simulink model "Aircraft6dof_forTrimAndLin_ATT_wInputs"  (R2023b)
settings: Solver=ode4  StartTime=startTime  StopTime=stopTime  FixedStep=stepTime  RelTol=1e-3  EnableMultiTasking=on
values from neighbouring files (symbols this model uses):
  a0_s2 = 0    [SetupForTrimAndLin_Aircraft6dof.m]
  a0_s3 = 0    [SetupForTrimAndLin_Aircraft6dof.m]
  a0_s4 = 0.05    [SetupForTrimAndLin_Aircraft6dof.m]
  a0_s5 = 0.05    [SetupForTrimAndLin_Aircraft6dof.m]
  AR_s2 = b_s2 / c_s2    [SetupForTrimAndLin_Aircraft6dof.m]
  AR_s3 = b_s3 / c_s3    [SetupForTrimAndLin_Aircraft6dof.m]
  AR_s4 = (b_s4+b_s5) / c_s4    [SetupForTrimAndLin_Aircraft6dof.m]
  AR_s5 = (b_s4+b_s5) / c_s5    [SetupForTrimAndLin_Aircraft6dof.m]
  c_s2 = componentMassesAndGeom(3,2)    [SetupForTrimAndLin_Aircraft6dof.m]
  c_s3 = componentMassesAndGeom(4,2)    [SetupForTrimAndLin_Aircraft6dof.m]
  c_s4 = componentMassesAndGeom(1,2)    [SetupForTrimAndLin_Aircraft6dof.m]
  c_s5 = componentMassesAndGeom(2,2)    [SetupForTrimAndLin_Aircraft6dof.m]
  CD0_s2 = 0.01    [SetupForTrimAndLin_Aircraft6dof.m]
  CD0_s3 = 0.01    [SetupForTrimAndLin_Aircraft6dof.m]
  CD0_s4 = 0.01    [SetupForTrimAndLin_Aircraft6dof.m]
  CD0_s5 = 0.01    [SetupForTrimAndLin_Aircraft6dof.m]
  CDa_s2 = 1    [SetupForTrimAndLin_Aircraft6dof.m]
  CDa_s3 = 1    [SetupForTrimAndLin_Aircraft6dof.m]
  CDa_s4 = 1    [SetupForTrimAndLin_Aircraft6dof.m]
  CDa_s5 = 1    [SetupForTrimAndLin_Aircraft6dof.m]
  CL0_s2 = 0    [SetupForTrimAndLin_Aircraft6dof.m]
  CL0_s3 = 0    [SetupForTrimAndLin_Aircraft6dof.m]
  CL0_s4 = 0.05    [SetupForTrimAndLin_Aircraft6dof.m]
  CL0_s5 = 0.05    [SetupForTrimAndLin_Aircraft6dof.m]
  CM0_s2 = 0    [SetupForTrimAndLin_Aircraft6dof.m]
  CM0_s3 = 0    [SetupForTrimAndLin_Aircraft6dof.m]
  CM0_s4 = -0.05    [SetupForTrimAndLin_Aircraft6dof.m]
  CM0_s5 = -0.05    [SetupForTrimAndLin_Aircraft6dof.m]
  CMa_s2 = 0    [SetupForTrimAndLin_Aircraft6dof.m]
  CMa_s3 = 0    [SetupForTrimAndLin_Aircraft6dof.m]
  CMa_s4 = 0    [SetupForTrimAndLin_Aircraft6dof.m]
  CMa_s5 = 0    [SetupForTrimAndLin_Aircraft6dof.m]
  dCL_du = 3    [SetupForTrimAndLin_Aircraft6dof.m]
  dE_0 = 0    [SetupForTrimAndLin_Aircraft6dof.m]
  dEL_0 = 0    [SetupForTrimAndLin_Aircraft6dof.m]
  dER_0 = 0    [SetupForTrimAndLin_Aircraft6dof.m]
  dR_0 = 0    [SetupForTrimAndLin_Aircraft6dof.m]
  e_s2 = 0.8    [SetupForTrimAndLin_Aircraft6dof.m]
  e_s3 = 0.8    [SetupForTrimAndLin_Aircraft6dof.m]
  e_s4 = 0.9    [SetupForTrimAndLin_Aircraft6dof.m]
  e_s5 = 0.9    [SetupForTrimAndLin_Aircraft6dof.m]
  g_E_N = [0; 0; 9.81]*1    [SetupAndRun_Aircraft6dof.m]    (also in SetupForTrimAndLin_Aircraft6dof.m = [0; 0; 9.81])
  i_s2 = -0.1    [SetupForTrimAndLin_Aircraft6dof.m]
  i_s3 = 0    [SetupForTrimAndLin_Aircraft6dof.m]
  i_s4 = 0.0    (= 0)    [SetupForTrimAndLin_Aircraft6dof.m]
  i_s5 = 0.0    (= 0)    [SetupForTrimAndLin_Aircraft6dof.m]
  InitAtt = InitAtt_deg * deg2rad    [SetupAndRun_Aircraft6dof.m]    (also in SetupForTrimAndLin_Aircraft6dof.m)
  InitPos = InitPos_deg .* [deg2rad; deg2rad; 1]    [SetupAndRun_Aircraft6dof.m]    (also in SetupForTrimAndLin_Aircraft6dof.m)
  InitRates = Rates_Trim    [SetupAndRun_Aircraft6dof.m]    (also in SetupForTrimAndLin_Aircraft6dof.m = [0; 0; 0])
  InitVel = Vel_B_BA_Trim    [SetupAndRun_Aircraft6dof.m]    (also in SetupForTrimAndLin_Aircraft6dof.m = [15; 0; 0])
  J = zeros(3,3)    [DefineAircraftGeometry.m]    (also in InitializeModel.m = ASW.RotationalInertiaMatrix; SetupAndRun_Aircraft6dof.m = [0.049 0 -0.0004; 0 0.022 0; -0.0004 0 0.071]; SetupForTrimAndLin_Aircraft6dof.m)
  m = sum(obj.componentMassesAndGeom(:,1))    [DefineAircraftGeometry.m]    (also in SetupForTrimAndLin_Aircraft6dof.m = sum(componentMassesAndGeom(:,1)))
  MixMatrix = [-1 1 0 0 ... (first row only)    [SetupForTrimAndLin_Aircraft6dof.m]
  n_s2 = [0; 0; -1]    [SetupForTrimAndLin_Aircraft6dof.m]
  n_s3 = [0; 1; 0]    [SetupForTrimAndLin_Aircraft6dof.m]
  n_s4 = [0; sin(0*pi/180);  -cos(0*pi/180)]    [SetupForTrimAndLin_Aircraft6dof.m]
  n_s5 = [0; sin(0*pi/180);  -cos(0*pi/180)]    [SetupForTrimAndLin_Aircraft6dof.m]
  om_motor_init = 0    [SetupForTrimAndLin_Aircraft6dof.m]
  omDot_motor = 0    [SetupForTrimAndLin_Aircraft6dof.m]
  S_s2 = c_s2 * b_s2    [SetupForTrimAndLin_Aircraft6dof.m]
  S_s3 = c_s3 * b_s3    [SetupForTrimAndLin_Aircraft6dof.m]
  S_s4 = c_s4 * b_s4    [SetupForTrimAndLin_Aircraft6dof.m]
  S_s5 = c_s5 * b_s5    [SetupForTrimAndLin_Aircraft6dof.m]
  S_u_s2 = c_u_s2*b_s2    [SetupForTrimAndLin_Aircraft6dof.m]
  S_u_s3 = c_u_s3*b_s3    [SetupForTrimAndLin_Aircraft6dof.m]
  S_u_s4 = c_u_s4*b_s4    [SetupForTrimAndLin_Aircraft6dof.m]
  S_u_s5 = c_u_s5*b_s5    [SetupForTrimAndLin_Aircraft6dof.m]
  tauE = 0.1    [SetupForTrimAndLin_Aircraft6dof.m]
  tauEL = 0.1    [SetupForTrimAndLin_Aircraft6dof.m]
  tauER = 0.1    [SetupForTrimAndLin_Aircraft6dof.m]
  tauR = 0.1    [SetupForTrimAndLin_Aircraft6dof.m]
  v_N_AE = [0; 0; 0]    [SetupAndRun_Aircraft6dof.m]    (also in SetupForTrimAndLin_Aircraft6dof.m)
  x_cm = sum(obj.componentMassesAndGeom(:,1) .* obj.componentMassesAndGeom(:,5:7)) / m    [DefineAircraftGeometry.m]    (also in SetupForTrimAndLin_Aircraft6dof.m = x_cm')
  x_s2 = [componentMassesAndGeom(3,5) + (1/4)*componentMassesAndGeom(3,2); componentMassesAndGeom(3,6);componentMassesAndGeom(3,7)]    [SetupForTrimAndLin_Aircraft6dof.m]
  x_s3 = [componentMassesAndGeom(4,5) + (1/4)*componentMassesAndGeom(4,2); componentMassesAndGeom(4,6);componentMassesAndGeom(4,7)]    [SetupForTrimAndLin_Aircraft6dof.m]
  x_s4 = [componentMassesAndGeom(1,5) + (1/4)*componentMassesAndGeom(1,2); componentMassesAndGeom(1,6);componentMassesAndGeom(1,7)]    [SetupForTrimAndLin_Aircraft6dof.m]
  x_s5 = [componentMassesAndGeom(2,5) + (1/4)*componentMassesAndGeom(2,2); componentMassesAndGeom(2,6);componentMassesAndGeom(2,7)]    [SetupForTrimAndLin_Aircraft6dof.m]
undefined symbols (not defined in the file or in its folder): InitQuat, J_int, n_int
libraries: vrlib x7, simulink x3
(part 1 of 2)
settings Model: Creator=McArthur  LastModifiedBy=prafulsigdel
settings SolverCC: AlgebraicLoopSolver=TrustRegion
settings DataIOCC: InitialState=[]  LimitDataPoints=on  LoadInitialState=on  SaveFormat=StructureWithTime  ReturnWorkspaceOutputs=off
settings OptimizationCC: DefaultParameterBehavior=Inlined  BufferReuse=off  LifeSpan=inf
settings DebuggingCC: UnconnectedInputMsg=warning  UnconnectedOutputMsg=warning  UnconnectedLineMsg=warning  InitInArrayFormatMsg=none  SFUnexpectedBacktrackingDiag=warning  SFNoUnconditionalDefaultTransitionDiag=warning  SFExecutionAtInitializationDiag=none  ArithmeticOperatorsInVariantConditions=warning
settings HardwareCC: ProdBitPerSizeT=32  ProdBitPerPtrDiffT=32  ProdWordSize=32  ProdHWDeviceType=Specified
settings ModelReferenceCC: PropagateSignalLabelsOutOfModel=off
settings SFSimCC: SimUseLocalCustomCode=off  CustomCodeUndefinedFunction=UseInterfaceOnly
settings RTWCC: RTWUseLocalCustomCode=off
settings CodeAppCC: StateflowObjectComments=on
settings GRTTargetCC: TargetLangStandard=C89/C90 (ANSI)
settings ConfigComp: CovMetricSettings=dw  CovSaveCumulativeToWorkspaceVar=on  CovSaveSingleToWorkspaceVar=on  CovExternalEMLEnable=off

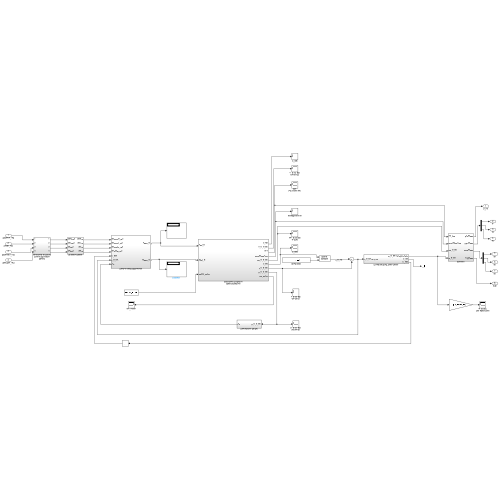
[thumbnail: Simulink's stored preview of the top-level diagram]
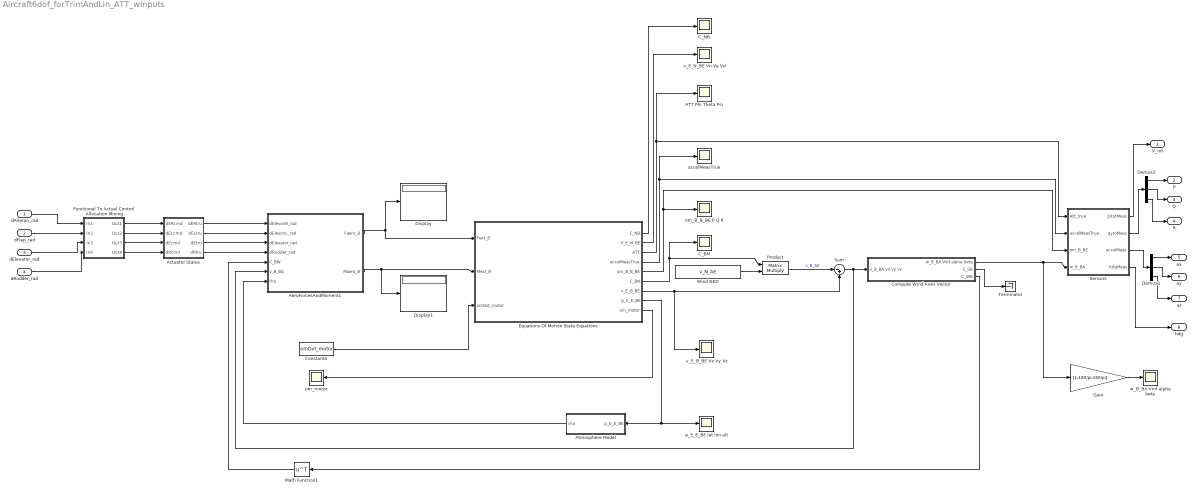
== system Aircraft6dof_forTrimAndLin_ATT_wInputs ==
  dAileron_rad : Inport
  dFlap_rad : Inport  Port=2
  dElevator_rad : Inport  Port=3
  dRudder_rad : Inport  Port=4
  ATT Phi Theta Psi : Scope
  Actuator States : Subsystem
  AeroForcesAndMoments : Subsystem
  Atmosphere Model : Subsystem
  C_BN : Scope
  C_NB : Scope
  Compute Wind Axes Vector : Subsystem
  Constant4 : Constant  Value=omDot_motor
  Demux1 : Demux  Outputs=3
  Demux2 : Demux  Outputs=3
  Display : Display
  Display1 : Display
  Equations Of Motion State Equations : Subsystem
  Functional To Actual Control Allocation Mixing : Subsystem
  Gain : Gain  Gain=[1;180/pi;180/pi]
  Math Function1 : Math  Operator=transpose  SignedPower=on
  Product : Product  Multiplication=Matrix(*)
  Sensors : Subsystem
  Sum : Sum  Inputs=|-+
  Terminator : Terminator
  Wind NED : Constant  Value=v_N_AE
  accelMeasTrue : Scope
  om_B_B_BE P Q R : Scope
  om_motor : Scope
  p_E_E_BE lat lon alt : Scope
  v_E_B_BE Vx Vy Vz : Scope
  v_E_N_BE Vn Ve Vd : Scope
  w_B_BA Vinf alpha beta : Scope
  V_inf : Outport
  P : Outport  Port=2
  Q : Outport  Port=3
  R : Outport  Port=4
  ax : Outport  Port=5
  ay : Outport  Port=6
  az : Outport  Port=7
  hdg : Outport  Port=8
  wires:
  Equations Of Motion State Equations/8(p_E_E_BE) -> Atmosphere Model/1(p_E_E_BE), p_E_E_BE lat lon alt/1
  Equations Of Motion State Equations/3(ATT) -> ATT Phi Theta Psi/1, Sensors/1(Att_true)
  AeroForcesAndMoments/2(Maero_B) -> Display1/1, Equations Of Motion State Equations/2(Mext_B)
  Constant4/1 -> Equations Of Motion State Equations/3(omDot_motor)
  AeroForcesAndMoments/1(Faero_B) -> Display/1, Equations Of Motion State Equations/1(Fext_B)
  Equations Of Motion State Equations/5(om_B_B_BE) -> Sensors/3(om_B_BE), om_B_B_BE P Q R/1
  Equations Of Motion State Equations/1(C_NB) -> C_NB/1
  Equations Of Motion State Equations/6(C_BN) -> C_BN/1, Product/1
  Equations Of Motion State Equations/7(v_E_B_BE) -> Sum/2, v_E_B_BE Vx Vy Vz/1
  Equations Of Motion State Equations/2(V_E_N_BE) -> v_E_N_BE Vn Ve Vd/1
  Compute Wind Axes Vector/1(w_B_BA Vinf alpha beta) -> Gain/1, Sensors/4(w_B_BA)
  Sum/1 -> AeroForcesAndMoments/6(v_B_BA), Compute Wind Axes Vector/1(v_B_BA vx vy vz)
  Product/1 -> Sum/1  "v_B_AE"
  Gain/1 -> w_B_BA Vinf alpha beta/1
  Equations Of Motion State Equations/9(om_motor) -> om_motor/1
  Atmosphere Model/1(rho) -> AeroForcesAndMoments/7(rho)
  Math Function1/1 -> AeroForcesAndMoments/5(C_BW)
  Compute Wind Axes Vector/3(C_WB) -> Math Function1/1
  Compute Wind Axes Vector/2(C_SB) -> Terminator/1
  Demux2/1 -> P/1
  Demux2/2 -> Q/1
  Demux2/3 -> R/1
  Sensors/1(pitotMeas) -> V_inf/1
  Sensors/2(gyroMeas) -> Demux2/1
  Equations Of Motion State Equations/4(accelMeasTrue) -> Sensors/2(accelMeasTrue), accelMeasTrue/1
  Wind NED/1 -> Product/2
  Demux1/1 -> ax/1
  Demux1/2 -> ay/1
  Demux1/3 -> az/1
  Sensors/3(accelMeas) -> Demux1/1
  Sensors/4(hdgMeas) -> hdg/1
  dAileron_rad/1 -> Functional To Actual Control Allocation Mixing/1(In1)
  dFlap_rad/1 -> Functional To Actual Control Allocation Mixing/2(In2)
  dElevator_rad/1 -> Functional To Actual Control Allocation Mixing/3(In3)
  dRudder_rad/1 -> Functional To Actual Control Allocation Mixing/4(In4)
  Functional To Actual Control Allocation Mixing/1(Out1) -> Actuator States/1(dERcmd)
  Functional To Actual Control Allocation Mixing/2(Out2) -> Actuator States/2(dELcmd)
  Functional To Actual Control Allocation Mixing/3(Out3) -> Actuator States/3(dEcmd)
  Functional To Actual Control Allocation Mixing/4(Out4) -> Actuator States/4(dRcmd)
  Actuator States/1(dERtru) -> AeroForcesAndMoments/1(dElevonR_rad)
  Actuator States/2(dELtru) -> AeroForcesAndMoments/2(dElevonL_rad)
  Actuator States/3(dEtru) -> AeroForcesAndMoments/3(dElevator_rad)
  Actuator States/4(dRtru) -> AeroForcesAndMoments/4(dRudder_rad)

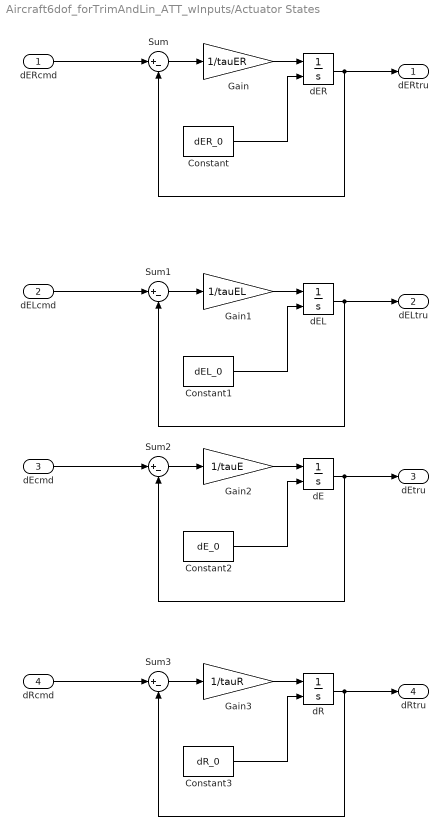
== system Aircraft6dof_forTrimAndLin_ATT_wInputs/Actuator States ==
  dERcmd : Inport
  dELcmd : Inport  Port=2
  dEcmd : Inport  Port=3
  dRcmd : Inport  Port=4
  Constant : Constant  Value=dER_0
  Constant1 : Constant  Value=dEL_0
  Constant2 : Constant  Value=dE_0
  Constant3 : Constant  Value=dR_0
  Gain : Gain  Gain=1/tauER
  Gain1 : Gain  Gain=1/tauEL
  Gain2 : Gain  Gain=1/tauE
  Gain3 : Gain  Gain=1/tauR
  Sum{,1..3} (4 alike) : Sum  Inputs=|+-
  dE : Integrator  InitialConditionSource=external
  dEL : Integrator  InitialConditionSource=external
  dER : Integrator  InitialConditionSource=external
  dR : Integrator  InitialConditionSource=external
  dERtru : Outport
  dELtru : Outport  Port=2
  dEtru : Outport  Port=3
  dRtru : Outport  Port=4
  wires:
  dER/1 -> Sum/2, dERtru/1
  dERcmd/1 -> Sum/1
  Gain/1 -> dER/1
  Sum/1 -> Gain/1
  Constant/1 -> dER/2
  dEL/1 -> Sum1/2, dELtru/1
  dELcmd/1 -> Sum1/1
  Gain1/1 -> dEL/1
  Sum1/1 -> Gain1/1
  Constant1/1 -> dEL/2
  dE/1 -> Sum2/2, dEtru/1
  dEcmd/1 -> Sum2/1
  Gain2/1 -> dE/1
  Sum2/1 -> Gain2/1
  Constant2/1 -> dE/2
  dR/1 -> Sum3/2, dRtru/1
  dRcmd/1 -> Sum3/1
  Gain3/1 -> dR/1
  Sum3/1 -> Gain3/1
  Constant3/1 -> dR/2

== system Aircraft6dof_forTrimAndLin_ATT_wInputs/AeroForcesAndMoments ==
  dElevonR_rad : Inport
  dElevonL_rad : Inport  Port=2
  dElevator_rad : Inport  Port=3
  dRudder_rad : Inport  Port=4
  C_BW : Inport  Port=5
  v_B_BA : Inport  Port=6
  rho : Inport  Port=7
  Add : Sum  Inputs=++++
  Add1 : Sum  Inputs=++++
  Display1 : Display
  Display3 : Display
  Surface2 : Subsystem
  Surface3 : Subsystem
  Surface4 : Subsystem
  Surface5 : Subsystem
  Faero_B : Outport
  Maero_B : Outport  Port=2
  wires:
  C_BW/1 -> Surface2/1(C_BW), Surface3/1(C_BW), Surface5/1(C_BW), Surface4/1(C_BW)
  v_B_BA/1 -> Surface3/2(v_B_BA), Surface2/2(v_B_BA), Surface5/2(v_B_BA), Surface4/2(v_B_BA)
  rho/1 -> Surface3/3(rho), Surface2/3(rho), Surface5/3(rho), Surface4/3(rho)
  Surface4/1(Fs4_B) -> Add/1
  Surface5/1(Fs5_B) -> Add/2
  Surface4/2(Ms4_B) -> Add1/1
  Surface5/2(Ms5_B) -> Add1/2
  Surface2/1(Fs2_B) -> Add/3
  Surface2/2(Ms2_B) -> Add1/3
  Add1/1 -> Display1/1, Maero_B/1
  Add/1 -> Display3/1, Faero_B/1
  Surface3/1(Fs2_B) -> Add/4
  Surface3/2(Ms2_B) -> Add1/4
  dElevonR_rad/1 -> Surface4/4(u_s#_rad)
  dElevonL_rad/1 -> Surface5/4(u_s#_rad)
  dElevator_rad/1 -> Surface2/4(u_s#_rad)
  dRudder_rad/1 -> Surface3/4(u_s#_rad)

== system Aircraft6dof_forTrimAndLin_ATT_wInputs/Atmosphere Model ==
  p_E_E_BE : Inport
  Compare To Constant : simulink/Logic and Bit Operations/Compare To Constant  relop=<=  const=11000  OutDataTypeStr=boolean
  Demux : Demux  Outputs=3
  Enhance Me Please! : Constant  Value=0
  Standard Atmosphere - Troposphere : MATLAB Function  TreatAsAtomicUnit=on
  Switch : Switch  Criteria=u2 ~= 0  Threshold=11000  SaturateOnIntegerOverflow=off  InputSameDT=off
  Terminator : Terminator
  Terminator1 : Terminator
  rho : Outport
  wires:
  p_E_E_BE/1 -> Demux/1
  Demux/1 -> Terminator/1
  Demux/2 -> Terminator1/1
  Demux/3 -> Standard Atmosphere - Troposphere/1(h), Compare To Constant/1
  Compare To Constant/1 -> Switch/2
  Standard Atmosphere - Troposphere/1(rho) -> Switch/1
  Switch/1 -> rho/1
  Enhance Me Please!/1 -> Switch/3

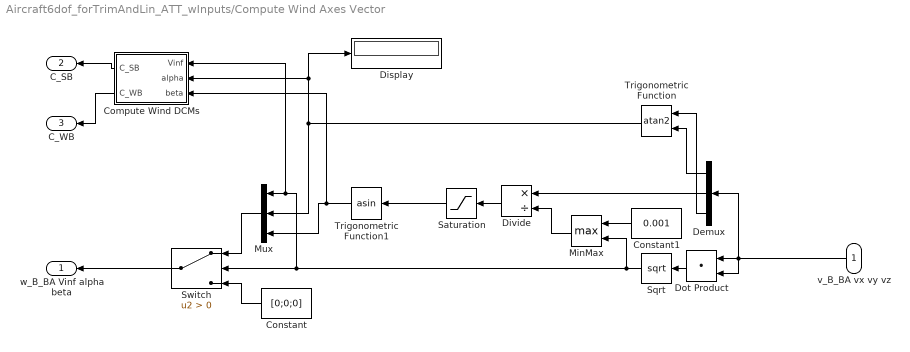
== system Aircraft6dof_forTrimAndLin_ATT_wInputs/Compute Wind Axes Vector ==
  v_B_BA vx vy vz : Inport
  Compute Wind DCMs : MATLAB Function  TreatAsAtomicUnit=on
  Constant : Constant  Value=[0;0;0]
  Constant1 : Constant  Value=0.001
  Demux : Demux  Outputs=3
  Display : Display
  Divide : Product  Inputs=*/
  Dot Product : DotProduct  OutDataTypeStr=Inherit: Inherit via internal rule
  MinMax : MinMax  Function=max  Inputs=2
  Mux : Mux  Inputs=3
  Saturation : Saturate  UpperLimit=1  LowerLimit=-1
  Sqrt : Sqrt
  Switch : Switch  Criteria=u2 > Threshold  SaturateOnIntegerOverflow=off  InputSameDT=off
  Trigonometric Function : Trigonometry  Operator=atan2
  Trigonometric Function1 : Trigonometry  Operator=asin
  w_B_BA Vinf alpha beta : Outport
  C_SB : Outport  Port=2
  C_WB : Outport  Port=3
  wires:
  Dot Product/1 -> Sqrt/1
  Mux/1 -> Switch/1
  Constant/1 -> Switch/3
  Trigonometric Function/1 -> Display/1, Compute Wind DCMs/2(alpha), Mux/2
  Switch/1 -> w_B_BA Vinf alpha beta/1
  Demux/3 -> Trigonometric Function/1
  v_B_BA vx vy vz/1 -> Demux/1, Dot Product/2, Dot Product/1
  Demux/1 -> Trigonometric Function/2
  Constant1/1 -> MinMax/1
  MinMax/1 -> Divide/2
  Demux/2 -> Divide/1
  Divide/1 -> Saturation/1
  Saturation/1 -> Trigonometric Function1/1
  Trigonometric Function1/1 -> Compute Wind DCMs/3(beta), Mux/3
  Sqrt/1 -> Compute Wind DCMs/1(Vinf), Mux/1, Switch/2, MinMax/2
  Compute Wind DCMs/2(C_WB) -> C_WB/1
  Compute Wind DCMs/1(C_SB) -> C_SB/1

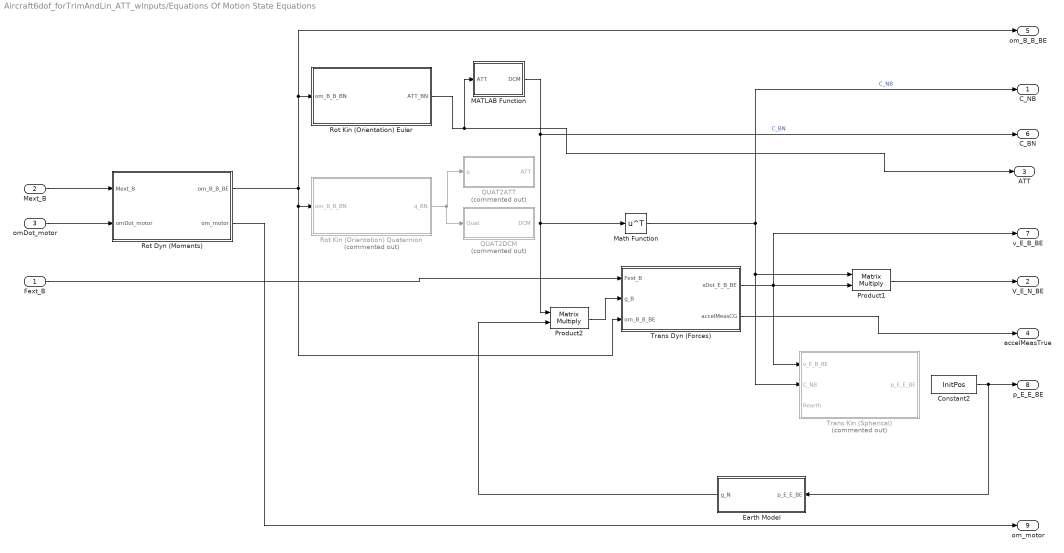
== system Aircraft6dof_forTrimAndLin_ATT_wInputs/Equations Of Motion State Equations ==
  Fext_B : Inport
  Mext_B : Inport  Port=2
  omDot_motor : Inport  Port=3
  Constant2 : Constant  Value=InitPos
  Earth Model : Subsystem
  MATLAB Function : MATLAB Function  TreatAsAtomicUnit=on
  Math Function : Math  Operator=transpose  SignedPower=on
  Product1 : Product  Multiplication=Matrix(*)
  Product2 : Product  Multiplication=Matrix(*)
  QUAT2ATT : Subsystem  Commented=on
  QUAT2DCM : Subsystem  Commented=on
  Rot Dyn (Moments) : Subsystem
  Rot Kin (Orientation) Euler : Subsystem
  Rot Kin (Orientation) Quaternion : Subsystem  Commented=on
  Trans Dyn (Forces) : Subsystem
  Trans Kin (Spherical) : Subsystem  Commented=on
  C_NB : Outport
  V_E_N_BE : Outport  Port=2
  ATT : Outport  Port=3
  accelMeasTrue : Outport  Port=4
  om_B_B_BE : Outport  Port=5
  C_BN : Outport  Port=6
  v_E_B_BE : Outport  Port=7
  p_E_E_BE : Outport  Port=8
  om_motor : Outport  Port=9
  wires:
  omDot_motor/1 -> Rot Dyn (Moments)/2(omDot_motor)
  Rot Dyn (Moments)/1(om_B_B_BE) -> Trans Dyn (Forces)/3(om_B_B_BE), Rot Kin (Orientation) Quaternion/1(om_B_B_BN), Rot Kin (Orientation) Euler/1(om_B_B_BN), om_B_B_BE/1
  Trans Dyn (Forces)/1(xDot_E_B_BE) -> Trans Kin (Spherical)/1(v_E_B_BE), v_E_B_BE/1, Product1/2
  Rot Kin (Orientation) Quaternion/1(q_BN) -> QUAT2DCM/1(Quat), QUAT2ATT/1(q)
  MATLAB Function/1(DCM) -> Math Function/1, Product2/1, C_BN/1  "C_BN"
  Mext_B/1 -> Rot Dyn (Moments)/1(Mext_B)
  Fext_B/1 -> Trans Dyn (Forces)/1(Fext_B)
  Rot Kin (Orientation) Euler/1(ATT_BN) -> ATT/1, MATLAB Function/1(ATT)
  Constant2/1 -> Earth Model/1(p_E_E_BE), p_E_E_BE/1
  Math Function/1 -> C_NB/1, Trans Kin (Spherical)/2(C_NB), Product1/1  "C_NB"
  Product1/1 -> V_E_N_BE/1
  Earth Model/1(g_N) -> Product2/2
  Product2/1 -> Trans Dyn (Forces)/2(g_B)
  Rot Dyn (Moments)/2(om_motor) -> om_motor/1
  Trans Dyn (Forces)/2(accelMeasCG) -> accelMeasTrue/1

== system Aircraft6dof_forTrimAndLin_ATT_wInputs/Functional To Actual Control Allocation Mixing ==
  In1 : Inport
  In2 : Inport  Port=2
  In3 : Inport  Port=3
  In4 : Inport  Port=4
  Constant1 : Constant  Value=MixMatrix
  Demux : Demux
  Mux : Mux
  Product1 : Product  Multiplication=Matrix(*)
  Out1 : Outport
  Out2 : Outport  Port=2
  Out3 : Outport  Port=3
  Out4 : Outport  Port=4
  wires:
  In1/1 -> Mux/1
  In2/1 -> Mux/2
  In3/1 -> Mux/3
  In4/1 -> Mux/4
  Demux/2 -> Out2/1
  Constant1/1 -> Product1/1
  Mux/1 -> Product1/2
  Demux/1 -> Out1/1
  Demux/4 -> Out4/1
  Demux/3 -> Out3/1
  Product1/1 -> Demux/1

== system Aircraft6dof_forTrimAndLin_ATT_wInputs/Sensors ==
  Att_true : Inport
  accelMeasTrue : Inport  Port=2
  om_B_BE : Inport  Port=3
  w_B_BA : Inport  Port=4
  Demux : Demux  Outputs=3
  Demux1 : Demux  Outputs=3
  Terminator{1..4} (4 alike) : Terminator
  pitotMeas : Outport
  gyroMeas : Outport  Port=2
  accelMeas : Outport  Port=3
  hdgMeas : Outport  Port=4
  wires:
  om_B_BE/1 -> gyroMeas/1
  w_B_BA/1 -> Demux/1
  Demux/3 -> Terminator1/1
  Demux/2 -> Terminator2/1
  Demux/1 -> pitotMeas/1
  accelMeasTrue/1 -> accelMeas/1
  Att_true/1 -> Demux1/1
  Demux1/1 -> Terminator3/1
  Demux1/2 -> Terminator4/1
  Demux1/3 -> hdgMeas/1

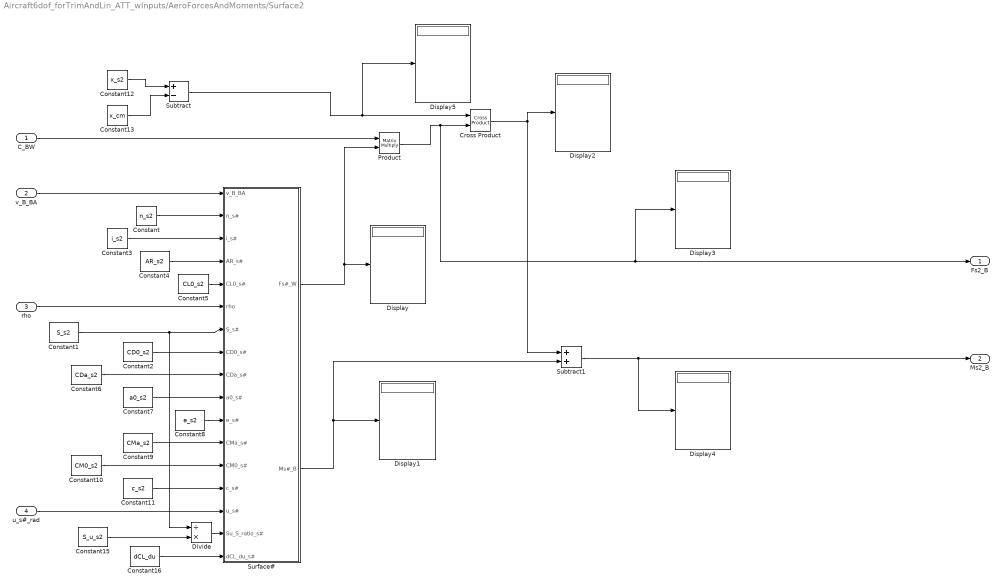
== system Aircraft6dof_forTrimAndLin_ATT_wInputs/AeroForcesAndMoments/Surface2 ==
  C_BW : Inport
  v_B_BA : Inport  Port=2
  rho : Inport  Port=3
  u_s#_rad : Inport  Port=4
  Constant : Constant  Value=n_s2
  Constant1 : Constant  Value=S_s2
  Constant10 : Constant  Value=CM0_s2
  Constant11 : Constant  Value=c_s2
  Constant12 : Constant  Value=x_s2
  Constant13 : Constant  Value=x_cm
  Constant15 : Constant  Value=S_u_s2
  Constant16 : Constant  Value=dCL_du
  Constant2 : Constant  Value=CD0_s2
  Constant3 : Constant  Value=i_s2
  Constant4 : Constant  Value=AR_s2
  Constant5 : Constant  Value=CL0_s2
  Constant6 : Constant  Value=CDa_s2
  Constant7 : Constant  Value=a0_s2
  Constant8 : Constant  Value=e_s2
  Constant9 : Constant  Value=CMa_s2
  Cross Product : vrlib/Utilities/Cross Product
  Display{,1..5} (6 alike) : Display
  Divide : Product  Inputs=/*
  Product : Product  Multiplication=Matrix(*)
  Subtract : Sum  Inputs=+-
  Subtract1 : Sum
  Surface# : Subsystem
  Fs2_B : Outport
  Ms2_B : Outport  Port=2
  wires:
  Subtract/1 -> Display5/1, Cross Product/1
  C_BW/1 -> Product/1
  Constant12/1 -> Subtract/1
  Constant13/1 -> Subtract/2
  Cross Product/1 -> Subtract1/1, Display2/1
  Product/1 -> Fs2_B/1, Display3/1, Cross Product/2
  Subtract1/1 -> Ms2_B/1, Display4/1
  Surface#/2(Ms#_B) -> Subtract1/2, Display1/1
  Constant10/1 -> Surface#/13(CM0_s#)
  Surface#/1(Fs#_W) -> Product/2, Display/1
  Constant11/1 -> Surface#/14(c_s#)
  Constant9/1 -> Surface#/12(CMa_s#)
  Constant7/1 -> Surface#/10(a0_s#)
  v_B_BA/1 -> Surface#/1(v_B_BA)
  Constant/1 -> Surface#/2(n_s#)
  Constant3/1 -> Surface#/3(i_s#)
  Constant4/1 -> Surface#/4(AR_s#)
  Constant5/1 -> Surface#/5(CL0_s#)
  rho/1 -> Surface#/6(rho)
  Constant2/1 -> Surface#/8(CD0_s#)
  Constant6/1 -> Surface#/9(CDa_s#)
  Constant8/1 -> Surface#/11(e_s#)
  Constant1/1 -> Divide/1, Surface#/7(S_s#)
  u_s#_rad/1 -> Surface#/15(u_s#)
  Constant15/1 -> Divide/2
  Constant16/1 -> Surface#/17(dCL_du_s#)
  Divide/1 -> Surface#/16(Su_S_ratio_s#)

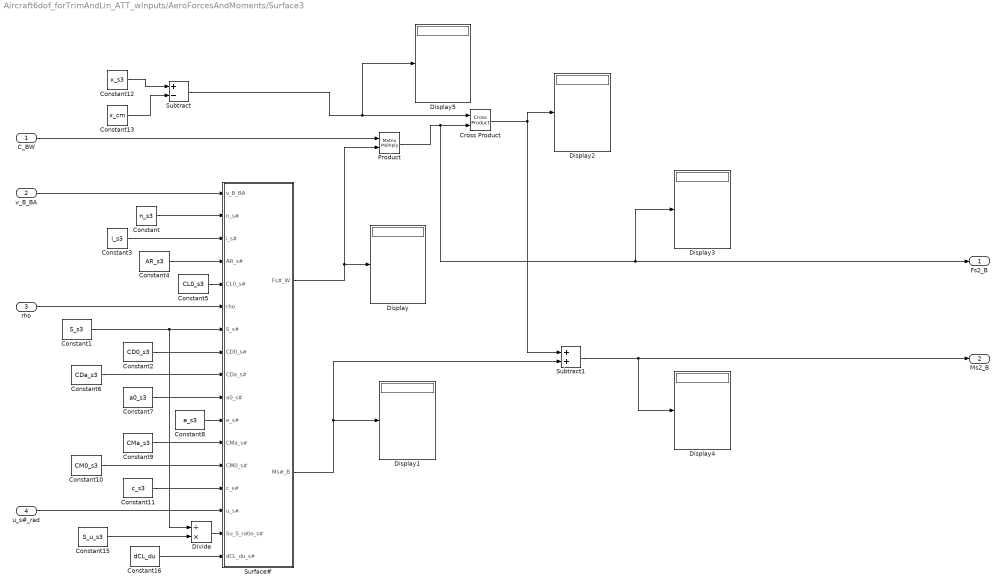
== system Aircraft6dof_forTrimAndLin_ATT_wInputs/AeroForcesAndMoments/Surface3 ==
  C_BW : Inport
  v_B_BA : Inport  Port=2
  rho : Inport  Port=3
  u_s#_rad : Inport  Port=4
  Constant : Constant  Value=n_s3
  Constant1 : Constant  Value=S_s3
  Constant10 : Constant  Value=CM0_s3
  Constant11 : Constant  Value=c_s3
  Constant12 : Constant  Value=x_s3
  Constant13 : Constant  Value=x_cm
  Constant15 : Constant  Value=S_u_s3
  Constant16 : Constant  Value=dCL_du
  Constant2 : Constant  Value=CD0_s3
  Constant3 : Constant  Value=i_s3
  Constant4 : Constant  Value=AR_s3
  Constant5 : Constant  Value=CL0_s3
  Constant6 : Constant  Value=CDa_s3
  Constant7 : Constant  Value=a0_s3
  Constant8 : Constant  Value=e_s3
  Constant9 : Constant  Value=CMa_s3
  Cross Product : vrlib/Utilities/Cross Product
  Display{,1..5} (6 alike) : Display
  Divide : Product  Inputs=/*
  Product : Product  Multiplication=Matrix(*)
  Subtract : Sum  Inputs=+-
  Subtract1 : Sum
  Surface# : Subsystem
  Fs2_B : Outport
  Ms2_B : Outport  Port=2
  wires:
  Subtract/1 -> Display5/1, Cross Product/1
  C_BW/1 -> Product/1
  Constant12/1 -> Subtract/1
  Constant13/1 -> Subtract/2
  Cross Product/1 -> Subtract1/1, Display2/1
  Product/1 -> Fs2_B/1, Display3/1, Cross Product/2
  Subtract1/1 -> Ms2_B/1, Display4/1
  Surface#/2(Ms#_B) -> Subtract1/2, Display1/1
  Constant10/1 -> Surface#/13(CM0_s#)
  Surface#/1(Fs#_W) -> Product/2, Display/1
  Constant11/1 -> Surface#/14(c_s#)
  Constant9/1 -> Surface#/12(CMa_s#)
  Constant7/1 -> Surface#/10(a0_s#)
  v_B_BA/1 -> Surface#/1(v_B_BA)
  Constant/1 -> Surface#/2(n_s#)
  Constant3/1 -> Surface#/3(i_s#)
  Constant4/1 -> Surface#/4(AR_s#)
  Constant5/1 -> Surface#/5(CL0_s#)
  rho/1 -> Surface#/6(rho)
  Constant2/1 -> Surface#/8(CD0_s#)
  Constant6/1 -> Surface#/9(CDa_s#)
  Constant8/1 -> Surface#/11(e_s#)
  Constant1/1 -> Divide/1, Surface#/7(S_s#)
  u_s#_rad/1 -> Surface#/15(u_s#)
  Constant15/1 -> Divide/2
  Constant16/1 -> Surface#/17(dCL_du_s#)
  Divide/1 -> Surface#/16(Su_S_ratio_s#)

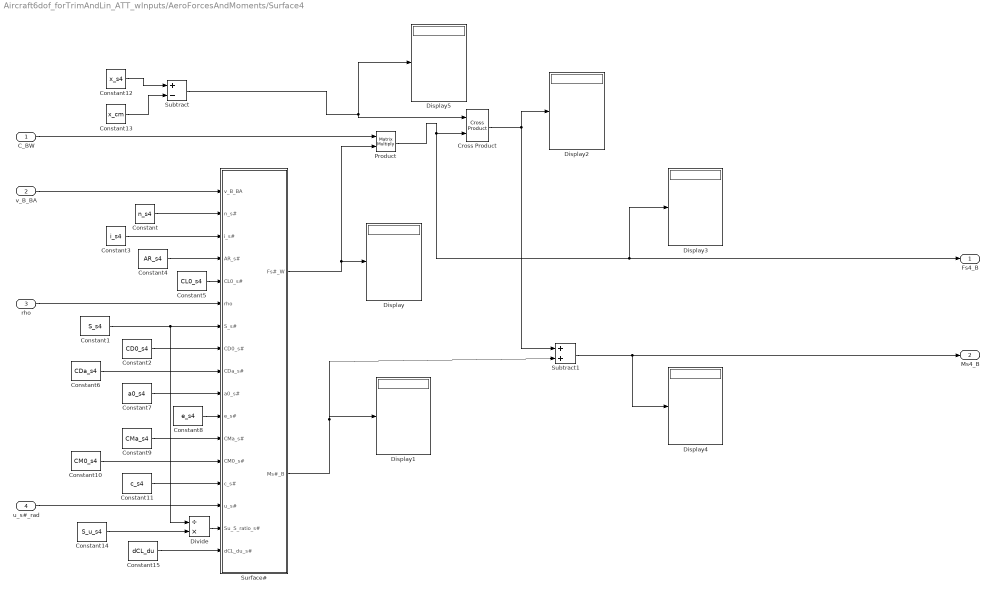
== system Aircraft6dof_forTrimAndLin_ATT_wInputs/AeroForcesAndMoments/Surface4 ==
  C_BW : Inport
  v_B_BA : Inport  Port=2
  rho : Inport  Port=3
  u_s#_rad : Inport  Port=4
  Constant : Constant  Value=n_s4
  Constant1 : Constant  Value=S_s4
  Constant10 : Constant  Value=CM0_s4
  Constant11 : Constant  Value=c_s4
  Constant12 : Constant  Value=x_s4
  Constant13 : Constant  Value=x_cm
  Constant14 : Constant  Value=S_u_s4
  Constant15 : Constant  Value=dCL_du
  Constant2 : Constant  Value=CD0_s4
  Constant3 : Constant  Value=i_s4
  Constant4 : Constant  Value=AR_s4
  Constant5 : Constant  Value=CL0_s4
  Constant6 : Constant  Value=CDa_s4
  Constant7 : Constant  Value=a0_s4
  Constant8 : Constant  Value=e_s4
  Constant9 : Constant  Value=CMa_s4
  Cross Product : vrlib/Utilities/Cross Product
  Display{,1..5} (6 alike) : Display
  Divide : Product  Inputs=/*
  Product : Product  Multiplication=Matrix(*)
  Subtract : Sum  Inputs=+-
  Subtract1 : Sum
  Surface# : Subsystem
  Fs4_B : Outport
  Ms4_B : Outport  Port=2
  wires:
  Subtract/1 -> Display5/1, Cross Product/1
  C_BW/1 -> Product/1
  Constant12/1 -> Subtract/1
  Constant13/1 -> Subtract/2
  Cross Product/1 -> Display2/1, Subtract1/1
  Product/1 -> Fs4_B/1, Display3/1, Cross Product/2
  Subtract1/1 -> Ms4_B/1, Display4/1
  Surface#/2(Ms#_B) -> Subtract1/2, Display1/1
  Constant10/1 -> Surface#/13(CM0_s#)
  Surface#/1(Fs#_W) -> Product/2, Display/1
  Constant11/1 -> Surface#/14(c_s#)
  Constant9/1 -> Surface#/12(CMa_s#)
  Constant7/1 -> Surface#/10(a0_s#)
  v_B_BA/1 -> Surface#/1(v_B_BA)
  Constant/1 -> Surface#/2(n_s#)
  Constant3/1 -> Surface#/3(i_s#)
  Constant4/1 -> Surface#/4(AR_s#)
  Constant5/1 -> Surface#/5(CL0_s#)
  rho/1 -> Surface#/6(rho)
  Constant1/1 -> Divide/1, Surface#/7(S_s#)
  Constant2/1 -> Surface#/8(CD0_s#)
  Constant6/1 -> Surface#/9(CDa_s#)
  Constant8/1 -> Surface#/11(e_s#)
  u_s#_rad/1 -> Surface#/15(u_s#)
  Divide/1 -> Surface#/16(Su_S_ratio_s#)
  Constant14/1 -> Divide/2
  Constant15/1 -> Surface#/17(dCL_du_s#)

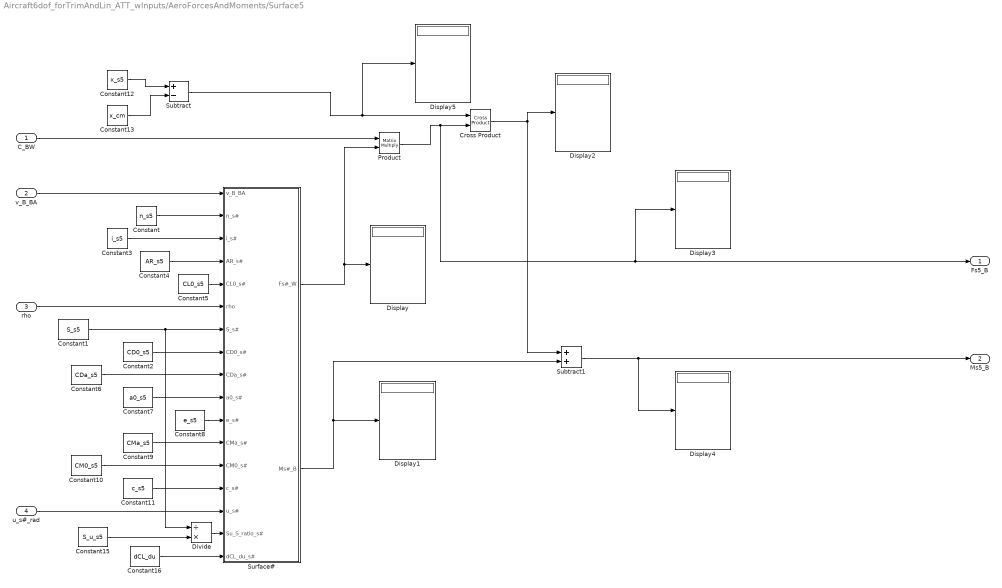
== system Aircraft6dof_forTrimAndLin_ATT_wInputs/AeroForcesAndMoments/Surface5 ==
  C_BW : Inport
  v_B_BA : Inport  Port=2
  rho : Inport  Port=3
  u_s#_rad : Inport  Port=4
  Constant : Constant  Value=n_s5
  Constant1 : Constant  Value=S_s5
  Constant10 : Constant  Value=CM0_s5
  Constant11 : Constant  Value=c_s5
  Constant12 : Constant  Value=x_s5
  Constant13 : Constant  Value=x_cm
  Constant15 : Constant  Value=S_u_s5
  Constant16 : Constant  Value=dCL_du
  Constant2 : Constant  Value=CD0_s5
  Constant3 : Constant  Value=i_s5
  Constant4 : Constant  Value=AR_s5
  Constant5 : Constant  Value=CL0_s5
  Constant6 : Constant  Value=CDa_s5
  Constant7 : Constant  Value=a0_s5
  Constant8 : Constant  Value=e_s5
  Constant9 : Constant  Value=CMa_s5
  Cross Product : vrlib/Utilities/Cross Product
  Display{,1..5} (6 alike) : Display
  Divide : Product  Inputs=/*
  Product : Product  Multiplication=Matrix(*)
  Subtract : Sum  Inputs=+-
  Subtract1 : Sum
  Surface# : Subsystem
  Fs5_B : Outport
  Ms5_B : Outport  Port=2
  wires:
  Constant8/1 -> Surface#/11(e_s#)
  Constant6/1 -> Surface#/9(CDa_s#)
  Constant2/1 -> Surface#/8(CD0_s#)
  rho/1 -> Surface#/6(rho)
  Constant5/1 -> Surface#/5(CL0_s#)
  Constant4/1 -> Surface#/4(AR_s#)
  Constant3/1 -> Surface#/3(i_s#)
  Constant/1 -> Surface#/2(n_s#)
  v_B_BA/1 -> Surface#/1(v_B_BA)
  Constant7/1 -> Surface#/10(a0_s#)
  Constant9/1 -> Surface#/12(CMa_s#)
  Constant11/1 -> Surface#/14(c_s#)
  Surface#/1(Fs#_W) -> Display/1, Product/2
  Constant10/1 -> Surface#/13(CM0_s#)
  Surface#/2(Ms#_B) -> Display1/1, Subtract1/2
  Subtract1/1 -> Display4/1, Ms5_B/1
  Product/1 -> Cross Product/2, Display3/1, Fs5_B/1
  Cross Product/1 -> Display2/1, Subtract1/1
  Constant13/1 -> Subtract/2
  Constant12/1 -> Subtract/1
  C_BW/1 -> Product/1
  Subtract/1 -> Cross Product/1, Display5/1
  Constant1/1 -> Surface#/7(S_s#), Divide/1
  u_s#_rad/1 -> Surface#/15(u_s#)
  Constant15/1 -> Divide/2
  Constant16/1 -> Surface#/17(dCL_du_s#)
  Divide/1 -> Surface#/16(Su_S_ratio_s#)

== system Aircraft6dof_forTrimAndLin_ATT_wInputs/Equations Of Motion State Equations/Earth Model ==
  p_E_E_BE : Inport
  Constant6 : Constant  Value=g_E_N
  Terminator : Terminator
  g_N : Outport
  wires:
  Constant6/1 -> g_N/1
  p_E_E_BE/1 -> Terminator/1

== system Aircraft6dof_forTrimAndLin_ATT_wInputs/Equations Of Motion State Equations/QUAT2ATT ==
  q : Inport
  Mux : Mux  Inputs=3
  Trigonometric Function1 : Trigonometry  Operator=atan2
  Trigonometric Function3 : Trigonometry  Operator=atan2
  fcn1 : Fcn  Expr=2*(u[2]*u[3] + u[1]*u[4])
  fcn2 : Fcn  Expr=u[1]*u[1] + u[2]*u[2] - u[3]*u[3] - u[4]*u[4]
  fcn3 : Fcn  Expr=-2*(u[2]*u[4] - u[1]*u[3])
  fcn4 : Fcn  Expr=2*(u[3]*u[4] + u[1]*u[2])
  fcn5 : Fcn  Expr=u[1]*u[1] - u[2]*u[2] - u[3]*u[3] + u[4]*u[4]
  trigFcn : Trigonometry  Operator=asin
  ATT : Outport
  wires:
  q/1 -> fcn2/1, fcn1/1, fcn4/1, fcn5/1, fcn3/1
  Trigonometric Function3/1 -> Mux/1  "psi"
  trigFcn/1 -> Mux/2  "theta"
  Trigonometric Function1/1 -> Mux/3  "phi"
  Mux/1 -> ATT/1
  fcn3/1 -> trigFcn/1
  fcn1/1 -> Trigonometric Function1/1
  fcn2/1 -> Trigonometric Function1/2
  fcn4/1 -> Trigonometric Function3/1
  fcn5/1 -> Trigonometric Function3/2

== system Aircraft6dof_forTrimAndLin_ATT_wInputs/Equations Of Motion State Equations/QUAT2DCM ==
  Quat : Inport  PortDimensions=4
  Subsystem : Subsystem
  Subsystem1 : Subsystem
  Subsystem2 : Subsystem
  Subsystem3 : Subsystem
  Subsystem4 : Subsystem
  Subsystem5 : Subsystem
  Subsystem6 : Subsystem
  Subsystem7 : Subsystem
  Subsystem8 : Subsystem
  Vector Concatenate : Concatenate  NumInputs=3
  Vector Concatenate1 : Concatenate  NumInputs=3
  Vector Concatenate2 : Concatenate  NumInputs=3
  Vector Concatenate3 : Concatenate  NumInputs=3  Mode=Multidimensional array  ConcatenateDimension=2
  norm : Subsystem
  DCM : Outport  PortDimensions=[3,3]  InitialOutput=0
  wires:
  Subsystem1/1(A12) -> Vector Concatenate1/1
  Subsystem7/1(A22) -> Vector Concatenate1/2
  norm/1(q/|q|) -> Subsystem/1(normal(q)), Subsystem8/1(normal(q)), Subsystem4/1(normal(q)), Subsystem2/1(normal(q)), Subsystem6/1(normal(q)), Subsystem7/1(normal(q)), Subsystem1/1(normal(q)), Subsystem5/1(normal(q)), Subsystem3/1(normal(q))
  Quat/1 -> norm/1(q)
  Subsystem8/1(A33) -> Vector Concatenate2/3
  Subsystem4/1(A23) -> Vector Concatenate2/2
  Subsystem2/1(A13) -> Vector Concatenate2/1
  Subsystem6/1(A32) -> Vector Concatenate1/3
  Subsystem5/1(A31) -> Vector Concatenate/3
  Subsystem3/1(A21) -> Vector Concatenate/2
  Subsystem/1(A11) -> Vector Concatenate/1
  Vector Concatenate3/1 -> DCM/1
  Vector Concatenate/1 -> Vector Concatenate3/1
  Vector Concatenate1/1 -> Vector Concatenate3/2
  Vector Concatenate2/1 -> Vector Concatenate3/3

== system Aircraft6dof_forTrimAndLin_ATT_wInputs/Equations Of Motion State Equations/Rot Dyn (Moments) ==
  Mext_B : Inport
  omDot_motor : Inport  Port=2
  Add : Sum  Inputs=+---
  Constant4 : Constant  Value=J
  Cross Product1 : vrlib/Utilities/Cross Product
  Integrate : Subsystem
  Internal Rotational Component 01 : Subsystem
  Product : Product  Multiplication=Matrix(*)
  Product1 : Product  Multiplication=Matrix(*)
  inv of matrix : MATLAB Function  TreatAsAtomicUnit=on
  om_B_B_BE : Outport
  om_motor : Outport  Port=2
  wires:
  Mext_B/1 -> Add/1
  Constant4/1 -> inv of matrix/1(u), Product/1
  Product/1 -> Cross Product1/2
  Cross Product1/1 -> Add/2
  inv of matrix/1(y) -> Product1/1
  Add/1 -> Product1/2
  omDot_motor/1 -> Internal Rotational Component 01/2(om_int_dot)
  Internal Rotational Component 01/1(hInt) -> Add/3
  Internal Rotational Component 01/2(hIntDot) -> Add/4
  Internal Rotational Component 01/3(om_motor) -> om_motor/1
  Integrate/1(om) -> Internal Rotational Component 01/1(om_B_B_BE), Cross Product1/1, Product/2, om_B_B_BE/1
  Product1/1 -> Integrate/1(omDot)

== system Aircraft6dof_forTrimAndLin_ATT_wInputs/Equations Of Motion State Equations/Rot Kin (Orientation) Euler ==
  om_B_B_BN : Inport
  Integrate : Subsystem
  MATLAB Function : MATLAB Function  TreatAsAtomicUnit=on
  Product : Product  Multiplication=Matrix(*)
  ATT_BN : Outport
  wires:
  om_B_B_BN/1 -> Product/2
  Product/1 -> Integrate/1(AttDot)
  Integrate/1(Att) -> MATLAB Function/1(ATT), ATT_BN/1
  MATLAB Function/1(MATRIX) -> Product/1

== system Aircraft6dof_forTrimAndLin_ATT_wInputs/Equations Of Motion State Equations/Rot Kin (Orientation) Quaternion ==
  om_B_B_BN : Inport
  Constant1 : Constant  Value=0
  Constant2 : Constant  Value=InitQuat
  Demux : Demux  Outputs=3
  Gain : Gain  Gain=1/2
  Mux : Mux
  QuatMult : Subsystem
  QuatStates : Integrator  InitialConditionSource=external
  norm1 : Subsystem
  q_BN : Outport
  wires:
  Constant2/1 -> QuatStates/2
  om_B_B_BN/1 -> Demux/1
  Demux/3 -> Mux/4
  Demux/2 -> Mux/3
  Demux/1 -> Mux/2
  Constant1/1 -> Mux/1
  Mux/1 -> QuatMult/2(r)
  QuatMult/1(q*r) -> Gain/1
  Gain/1 -> QuatStates/1
  QuatStates/1 -> norm1/1(q)
  norm1/1(q/|q|) -> QuatMult/1(q), q_BN/1

== system Aircraft6dof_forTrimAndLin_ATT_wInputs/Equations Of Motion State Equations/Trans Dyn (Forces) ==
  Fext_B : Inport
  g_B : Inport  Port=2
  om_B_B_BE : Inport  Port=3
  Add : Sum  Inputs=++-
  Constant4 : Constant  Value=m
  Cross Product : vrlib/Utilities/Cross Product
  Display{,1..4} (5 alike) : Display
  Divide2 : Product  Inputs=*/
  Integrate : Subsystem
  xDot_E_B_BE : Outport
  accelMeasCG : Outport  Port=2
  wires:
  Add/1 -> Integrate/1(VelDot), Display/1  "xDotDot_E_B_BE"
  g_B/1 -> Display3/1, Add/2  "g_B"
  Fext_B/1 -> Divide2/1
  Constant4/1 -> Divide2/2
  Divide2/1 -> accelMeasCG/1, Display2/1, Add/1
  om_B_B_BE/1 -> Cross Product/1
  Integrate/1(Vel) -> Cross Product/2, Display1/1, xDot_E_B_BE/1
  Cross Product/1 -> Display4/1, Add/3

== system Aircraft6dof_forTrimAndLin_ATT_wInputs/Equations Of Motion State Equations/Trans Kin (Spherical) ==
  v_E_B_BE : Inport
  C_NB : Inport  Port=2
  Rearth : Inport  Port=3
  AltDot : Gain  Gain=-1
  Constant2 : Constant  Value=InitPos
  Demux : Demux  Outputs=3
  Demux1 : Demux  Outputs=3
  Demux2 : Demux  Outputs=3
  LatDot : Subsystem
  LonDot : Subsystem
  Mux : Mux  Inputs=3
  Mux1 : Mux  Inputs=3
  PositionStates : Integrator  InitialConditionSource=external
  Product : Product  Multiplication=Matrix(*)
  Terminator : Terminator
  bound lat : Saturate  UpperLimit=pi/2  LowerLimit=-pi/2
  wrap lon : Subsystem
  p_E_E_BE : Outport
  wires:
  Mux1/1 -> p_E_E_BE/1, Demux1/1
  Product/1 -> Demux/1
  Rearth/1 -> LatDot/2(Rearth), LonDot/2(Rearth)
  Demux1/3 -> LatDot/3(alt), LonDot/3(alt)
  Demux/3 -> AltDot/1
  AltDot/1 -> Mux/3
  Mux/1 -> PositionStates/1
  Constant2/1 -> PositionStates/2
  Demux1/2 -> Terminator/1
  PositionStates/1 -> Demux2/1
  Demux2/1 -> bound lat/1
  bound lat/1 -> Mux1/1
  Demux2/3 -> Mux1/3
  Demux2/2 -> wrap lon/1(lon)
  wrap lon/1(-pi < lon <= pi) -> Mux1/2
  C_NB/1 -> Product/1
  v_E_B_BE/1 -> Product/2
  Demux/1 -> LatDot/1(Vn)
  LatDot/1(latDot) -> Mux/1
  Demux/2 -> LonDot/1(Ve)
  Demux1/1 -> LonDot/4(lat)
  LonDot/1(lonDot) -> Mux/2

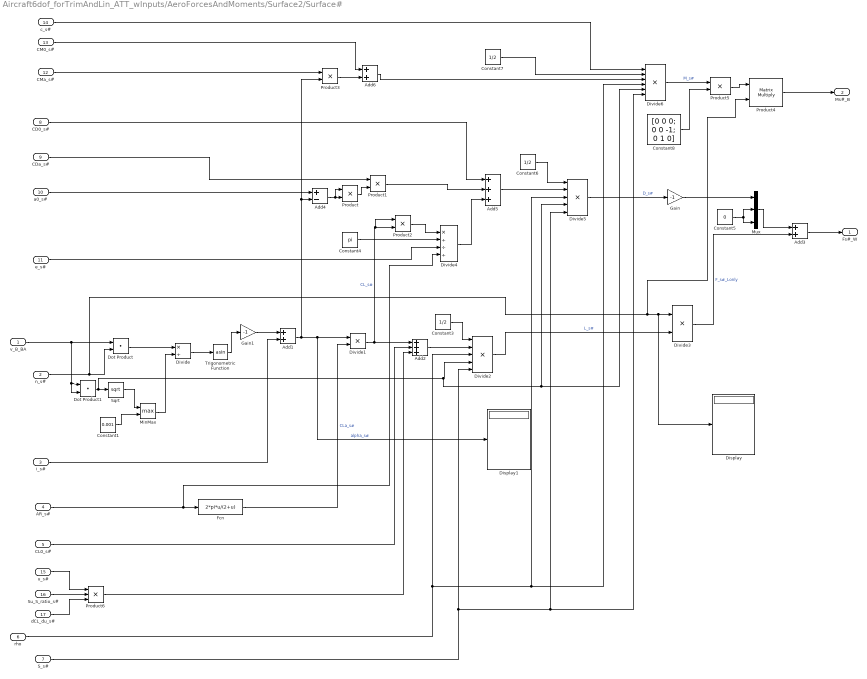
== system Aircraft6dof_forTrimAndLin_ATT_wInputs/AeroForcesAndMoments/Surface2/Surface# ==
  v_B_BA : Inport
  n_s# : Inport  Port=2
  i_s# : Inport  Port=3
  AR_s# : Inport  Port=4
  CL0_s# : Inport  Port=5
  rho : Inport  Port=6
  S_s# : Inport  Port=7
  CD0_s# : Inport  Port=8
  CDa_s# : Inport  Port=9
  a0_s# : Inport  Port=10
  e_s# : Inport  Port=11
  CMa_s# : Inport  Port=12
  CM0_s# : Inport  Port=13
  c_s# : Inport  Port=14
  u_s# : Inport  Port=15
  Su_S_ratio_s# : Inport  Port=16
  dCL_du_s# : Inport  Port=17
  Add1 : Sum
  Add2 : Sum  Inputs=+++
  Add3 : Sum
  Add4 : Sum  Inputs=+-
  Add5 : Sum  Inputs=+++
  Add6 : Sum
  Constant1 : Constant  Value=0.001
  Constant3 : Constant  Value=1/2
  Constant4 : Constant  Value=pi
  Constant5 : Constant  Value=0
  Constant6 : Constant  Value=1/2
  Constant7 : Constant  Value=1/2
  Constant8 : Constant  Value=[0 0 0; 0 0 -1; 0 1 0]
  Display : Display
  Display1 : Display
  Divide : Product  Inputs=*/
  Divide1 : Product  Inputs=**
  Divide2 : Product  Inputs=*****
  Divide3 : Product  Inputs=**
  Divide4 : Product  Inputs=*///
  Divide5 : Product  Inputs=*****
  Divide6 : Product  Inputs=******
  Dot Product : DotProduct  OutDataTypeStr=Inherit: Inherit via internal rule
  Dot Product1 : DotProduct  OutDataTypeStr=Inherit: Inherit via internal rule
  Fcn : Fcn  Expr=2*pi*u/(2+u)
  Gain : Gain  Gain=-1
  Gain1 : Gain  Gain=-1
  MinMax : MinMax  Function=max  Inputs=2
  Mux : Mux  Inputs=3
  Product{,1..3,5} (5 alike) : Product
  Product4 : Product  Multiplication=Matrix(*)
  Product6 : Product  Inputs=3
  Sqrt : Sqrt
  Trigonometric Function : Trigonometry  Operator=asin
  Fs#_W : Outport
  Ms#_B : Outport  Port=2
  wires:
  v_B_BA/1 -> Dot Product1/1, Dot Product1/2, Dot Product/1
  n_s#/1 -> Product4/2, Display/1, Divide3/1, Dot Product/2
  Dot Product/1 -> Divide/1
  Constant1/1 -> MinMax/2
  MinMax/1 -> Divide/2
  Sqrt/1 -> MinMax/1
  Divide/1 -> Trigonometric Function/1
  i_s#/1 -> Add1/2
  Add1/1 -> Product3/2, Add4/2, Display1/1, Divide1/1  "alpha_s#"
  AR_s#/1 -> Divide4/4, Fcn/1
  Fcn/1 -> Divide1/2  "CLa_s#"
  Divide1/1 -> Product2/1, Product2/2, Add2/1  "CL_s#"
  CL0_s#/1 -> Add2/2
  Add2/1 -> Divide2/2
  Constant3/1 -> Divide2/1
  Divide2/1 -> Divide3/2  "L_s#"
  Divide3/1 -> Add3/2  "F_s#_Lonly"
  Mux/1 -> Add3/1
  a0_s#/1 -> Add4/1
  Add4/1 -> Product/1, Product/2
  Product/1 -> Product1/2
  CDa_s#/1 -> Product1/1
  Product2/1 -> Divide4/1
  Constant4/1 -> Divide4/2
  e_s#/1 -> Divide4/3
  Divide4/1 -> Add5/3
  Product1/1 -> Add5/2
  CD0_s#/1 -> Add5/1
  Add5/1 -> Divide5/2
  Constant5/1 -> Mux/2, Mux/3
  CMa_s#/1 -> Product3/1
  CM0_s#/1 -> Add6/1
  Product3/1 -> Add6/2
  Constant6/1 -> Divide5/1
  Divide5/1 -> Gain/1  "D_s#"
  Dot Product1/1 -> Divide6/5, Divide5/4, Divide2/4, Sqrt/1
  rho/1 -> Divide6/4, Divide5/3, Divide2/3
  S_s#/1 -> Divide6/6, Divide5/5, Divide2/5
  Add6/1 -> Divide6/3
  Constant7/1 -> Divide6/2
  c_s#/1 -> Divide6/1
  Add3/1 -> Fs#_W/1
  Divide6/1 -> Product5/1  "M_s#"
  Constant8/1 -> Product5/2
  Product4/1 -> Ms#_B/1
  Product5/1 -> Product4/1
  Gain/1 -> Mux/1
  Gain1/1 -> Add1/1
  Trigonometric Function/1 -> Gain1/1
  u_s#/1 -> Product6/1
  Su_S_ratio_s#/1 -> Product6/2
  dCL_du_s#/1 -> Product6/3
  Product6/1 -> Add2/3

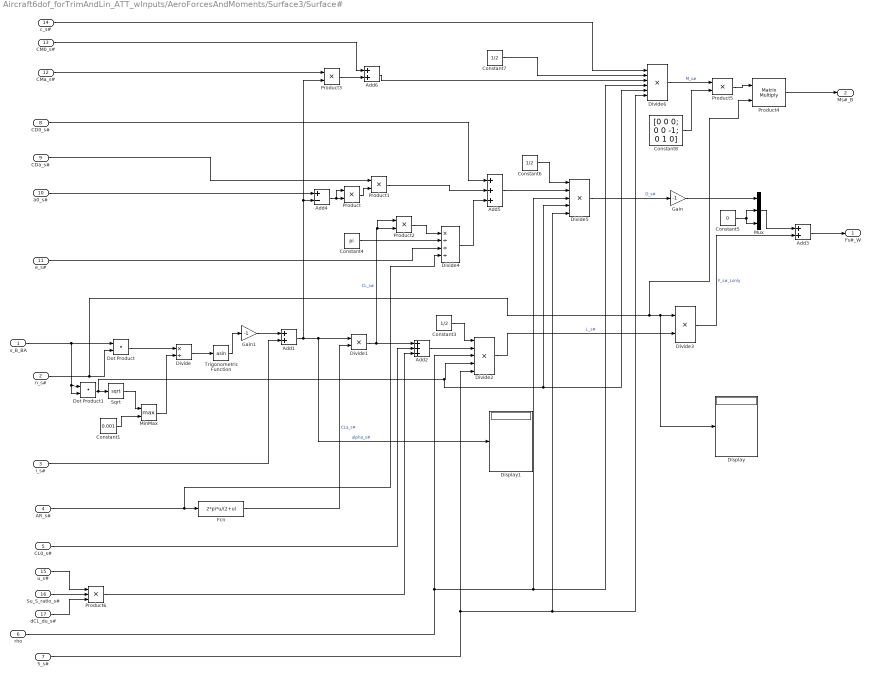
== system Aircraft6dof_forTrimAndLin_ATT_wInputs/AeroForcesAndMoments/Surface3/Surface# ==
  v_B_BA : Inport
  n_s# : Inport  Port=2
  i_s# : Inport  Port=3
  AR_s# : Inport  Port=4
  CL0_s# : Inport  Port=5
  rho : Inport  Port=6
  S_s# : Inport  Port=7
  CD0_s# : Inport  Port=8
  CDa_s# : Inport  Port=9
  a0_s# : Inport  Port=10
  e_s# : Inport  Port=11
  CMa_s# : Inport  Port=12
  CM0_s# : Inport  Port=13
  c_s# : Inport  Port=14
  u_s# : Inport  Port=15
  Su_S_ratio_s# : Inport  Port=16
  dCL_du_s# : Inport  Port=17
  Add1 : Sum
  Add2 : Sum  Inputs=+++
  Add3 : Sum
  Add4 : Sum  Inputs=+-
  Add5 : Sum  Inputs=+++
  Add6 : Sum
  Constant1 : Constant  Value=0.001
  Constant3 : Constant  Value=1/2
  Constant4 : Constant  Value=pi
  Constant5 : Constant  Value=0
  Constant6 : Constant  Value=1/2
  Constant7 : Constant  Value=1/2
  Constant8 : Constant  Value=[0 0 0; 0 0 -1; 0 1 0]
  Display : Display
  Display1 : Display
  Divide : Product  Inputs=*/
  Divide1 : Product  Inputs=**
  Divide2 : Product  Inputs=*****
  Divide3 : Product  Inputs=**
  Divide4 : Product  Inputs=*///
  Divide5 : Product  Inputs=*****
  Divide6 : Product  Inputs=******
  Dot Product : DotProduct  OutDataTypeStr=Inherit: Inherit via internal rule
  Dot Product1 : DotProduct  OutDataTypeStr=Inherit: Inherit via internal rule
  Fcn : Fcn  Expr=2*pi*u/(2+u)
  Gain : Gain  Gain=-1
  Gain1 : Gain  Gain=-1
  MinMax : MinMax  Function=max  Inputs=2
  Mux : Mux  Inputs=3
  Product{,1..3,5} (5 alike) : Product
  Product4 : Product  Multiplication=Matrix(*)
  Product6 : Product  Inputs=3
  Sqrt : Sqrt
  Trigonometric Function : Trigonometry  Operator=asin
  Fs#_W : Outport
  Ms#_B : Outport  Port=2
  wires:
  v_B_BA/1 -> Dot Product1/1, Dot Product1/2, Dot Product/1
  n_s#/1 -> Product4/2, Display/1, Divide3/1, Dot Product/2
  Dot Product/1 -> Divide/1
  Constant1/1 -> MinMax/2
  MinMax/1 -> Divide/2
  Sqrt/1 -> MinMax/1
  Divide/1 -> Trigonometric Function/1
  i_s#/1 -> Add1/2
  Add1/1 -> Product3/2, Add4/2, Display1/1, Divide1/1  "alpha_s#"
  AR_s#/1 -> Divide4/4, Fcn/1
  Fcn/1 -> Divide1/2  "CLa_s#"
  Divide1/1 -> Product2/1, Product2/2, Add2/1  "CL_s#"
  CL0_s#/1 -> Add2/2
  Add2/1 -> Divide2/2
  Constant3/1 -> Divide2/1
  Divide2/1 -> Divide3/2  "L_s#"
  Divide3/1 -> Add3/2  "F_s#_Lonly"
  Mux/1 -> Add3/1
  a0_s#/1 -> Add4/1
  Add4/1 -> Product/1, Product/2
  Product/1 -> Product1/2
  CDa_s#/1 -> Product1/1
  Product2/1 -> Divide4/1
  Constant4/1 -> Divide4/2
  e_s#/1 -> Divide4/3
  Divide4/1 -> Add5/3
  Product1/1 -> Add5/2
  CD0_s#/1 -> Add5/1
  Add5/1 -> Divide5/2
  Constant5/1 -> Mux/2, Mux/3
  CMa_s#/1 -> Product3/1
  CM0_s#/1 -> Add6/1
  Product3/1 -> Add6/2
  Constant6/1 -> Divide5/1
  Divide5/1 -> Gain/1  "D_s#"
  Dot Product1/1 -> Divide6/5, Divide5/4, Divide2/4, Sqrt/1
  rho/1 -> Divide6/4, Divide5/3, Divide2/3
  S_s#/1 -> Divide6/6, Divide5/5, Divide2/5
  Add6/1 -> Divide6/3
  Constant7/1 -> Divide6/2
  c_s#/1 -> Divide6/1
  Add3/1 -> Fs#_W/1
  Divide6/1 -> Product5/1  "M_s#"
  Constant8/1 -> Product5/2
  Product4/1 -> Ms#_B/1
  Product5/1 -> Product4/1
  Gain/1 -> Mux/1
  Gain1/1 -> Add1/1
  Trigonometric Function/1 -> Gain1/1
  u_s#/1 -> Product6/1
  Su_S_ratio_s#/1 -> Product6/2
  dCL_du_s#/1 -> Product6/3
  Product6/1 -> Add2/3

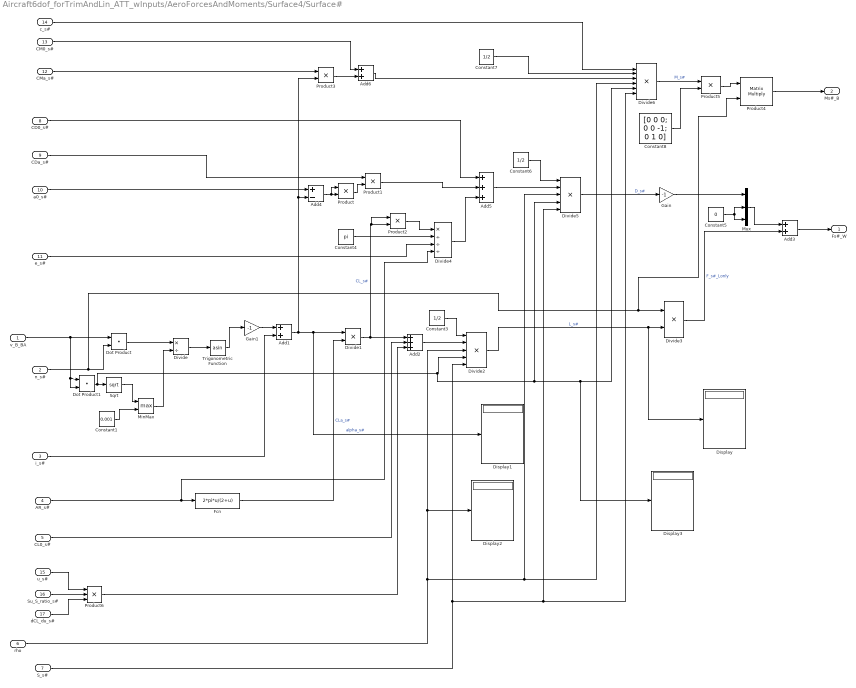
== system Aircraft6dof_forTrimAndLin_ATT_wInputs/AeroForcesAndMoments/Surface4/Surface# ==
  v_B_BA : Inport
  n_s# : Inport  Port=2
  i_s# : Inport  Port=3
  AR_s# : Inport  Port=4
  CL0_s# : Inport  Port=5
  rho : Inport  Port=6
  S_s# : Inport  Port=7
  CD0_s# : Inport  Port=8
  CDa_s# : Inport  Port=9
  a0_s# : Inport  Port=10
  e_s# : Inport  Port=11
  CMa_s# : Inport  Port=12
  CM0_s# : Inport  Port=13
  c_s# : Inport  Port=14
  u_s# : Inport  Port=15
  Su_S_ratio_s# : Inport  Port=16
  dCL_du_s# : Inport  Port=17
  Add1 : Sum
  Add2 : Sum  Inputs=+++
  Add3 : Sum
  Add4 : Sum  Inputs=+-
  Add5 : Sum  Inputs=+++
  Add6 : Sum
  Constant1 : Constant  Value=0.001
  Constant3 : Constant  Value=1/2
  Constant4 : Constant  Value=pi
  Constant5 : Constant  Value=0
  Constant6 : Constant  Value=1/2
  Constant7 : Constant  Value=1/2
  Constant8 : Constant  Value=[0 0 0; 0 0 -1; 0 1 0]
  Display{,1..3} (4 alike) : Display
  Divide : Product  Inputs=*/
  Divide1 : Product  Inputs=**
  Divide2 : Product  Inputs=*****
  Divide3 : Product  Inputs=**
  Divide4 : Product  Inputs=*///
  Divide5 : Product  Inputs=*****
  Divide6 : Product  Inputs=******
  Dot Product : DotProduct  OutDataTypeStr=Inherit: Inherit via internal rule
  Dot Product1 : DotProduct  OutDataTypeStr=Inherit: Inherit via internal rule
  Fcn : Fcn  Expr=2*pi*u/(2+u)
  Gain : Gain  Gain=-1
  Gain1 : Gain  Gain=-1
  MinMax : MinMax  Function=max  Inputs=2
  Mux : Mux  Inputs=3
  Product{,1..3,5} (5 alike) : Product
  Product4 : Product  Multiplication=Matrix(*)
  Product6 : Product  Inputs=3
  Sqrt : Sqrt
  Trigonometric Function : Trigonometry  Operator=asin
  Fs#_W : Outport
  Ms#_B : Outport  Port=2
  wires:
  v_B_BA/1 -> Dot Product1/1, Dot Product1/2, Dot Product/1
  n_s#/1 -> Product4/2, Divide3/1, Dot Product/2
  Dot Product/1 -> Divide/1
  Constant1/1 -> MinMax/2
  MinMax/1 -> Divide/2
  Sqrt/1 -> MinMax/1
  Divide/1 -> Trigonometric Function/1
  Gain1/1 -> Add1/1
  i_s#/1 -> Add1/2
  Add1/1 -> Product3/2, Add4/2, Display1/1, Divide1/1  "alpha_s#"
  AR_s#/1 -> Divide4/4, Fcn/1
  Fcn/1 -> Divide1/2  "CLa_s#"
  Divide1/1 -> Product2/1, Product2/2, Add2/1  "CL_s#"
  CL0_s#/1 -> Add2/2
  Add2/1 -> Divide2/2
  Constant3/1 -> Divide2/1
  Divide2/1 -> Display/1, Divide3/2  "L_s#"
  Divide3/1 -> Add3/2  "F_s#_Lonly"
  Mux/1 -> Add3/1
  a0_s#/1 -> Add4/1
  Add4/1 -> Product/1, Product/2
  Product/1 -> Product1/2
  CDa_s#/1 -> Product1/1
  Product2/1 -> Divide4/1
  Constant4/1 -> Divide4/2
  e_s#/1 -> Divide4/3
  Divide4/1 -> Add5/3
  Product1/1 -> Add5/2
  CD0_s#/1 -> Add5/1
  Add5/1 -> Divide5/2
  Constant5/1 -> Mux/2, Mux/3
  CMa_s#/1 -> Product3/1
  CM0_s#/1 -> Add6/1
  Product3/1 -> Add6/2
  Constant6/1 -> Divide5/1
  Divide5/1 -> Gain/1  "D_s#"
  Dot Product1/1 -> Display3/1, Divide6/5, Divide5/4, Divide2/4, Sqrt/1
  rho/1 -> Divide6/4, Divide5/3, Display2/1, Divide2/3
  S_s#/1 -> Divide6/6, Divide5/5, Divide2/5
  Add6/1 -> Divide6/3
  Constant7/1 -> Divide6/2
  c_s#/1 -> Divide6/1
  Add3/1 -> Fs#_W/1
  Divide6/1 -> Product5/1  "M_s#"
  Constant8/1 -> Product5/2
  Product4/1 -> Ms#_B/1
  Product5/1 -> Product4/1
  Gain/1 -> Mux/1
  Trigonometric Function/1 -> Gain1/1
  u_s#/1 -> Product6/1
  Su_S_ratio_s#/1 -> Product6/2
  dCL_du_s#/1 -> Product6/3
  Product6/1 -> Add2/3

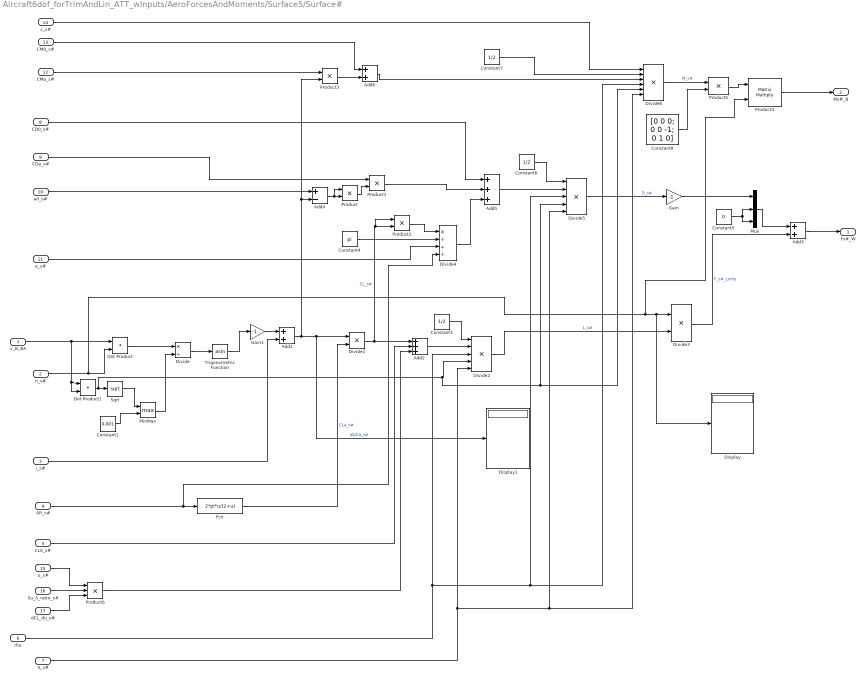
== system Aircraft6dof_forTrimAndLin_ATT_wInputs/AeroForcesAndMoments/Surface5/Surface# ==
  v_B_BA : Inport
  n_s# : Inport  Port=2
  i_s# : Inport  Port=3
  AR_s# : Inport  Port=4
  CL0_s# : Inport  Port=5
  rho : Inport  Port=6
  S_s# : Inport  Port=7
  CD0_s# : Inport  Port=8
  CDa_s# : Inport  Port=9
  a0_s# : Inport  Port=10
  e_s# : Inport  Port=11
  CMa_s# : Inport  Port=12
  CM0_s# : Inport  Port=13
  c_s# : Inport  Port=14
  u_s# : Inport  Port=15
  Su_S_ratio_s# : Inport  Port=16
  dCL_du_s# : Inport  Port=17
  Add1 : Sum
  Add2 : Sum  Inputs=+++
  Add3 : Sum
  Add4 : Sum  Inputs=+-
  Add5 : Sum  Inputs=+++
  Add6 : Sum
  Constant1 : Constant  Value=0.001
  Constant3 : Constant  Value=1/2
  Constant4 : Constant  Value=pi
  Constant5 : Constant  Value=0
  Constant6 : Constant  Value=1/2
  Constant7 : Constant  Value=1/2
  Constant8 : Constant  Value=[0 0 0; 0 0 -1; 0 1 0]
  Display : Display
  Display1 : Display
  Divide : Product  Inputs=*/
  Divide1 : Product  Inputs=**
  Divide2 : Product  Inputs=*****
  Divide3 : Product  Inputs=**
  Divide4 : Product  Inputs=*///
  Divide5 : Product  Inputs=*****
  Divide6 : Product  Inputs=******
  Dot Product : DotProduct  OutDataTypeStr=Inherit: Inherit via internal rule
  Dot Product1 : DotProduct  OutDataTypeStr=Inherit: Inherit via internal rule
  Fcn : Fcn  Expr=2*pi*u/(2+u)
  Gain : Gain  Gain=-1
  Gain1 : Gain  Gain=-1
  MinMax : MinMax  Function=max  Inputs=2
  Mux : Mux  Inputs=3
  Product{,1..3,5} (5 alike) : Product
  Product4 : Product  Multiplication=Matrix(*)
  Product6 : Product  Inputs=3
  Sqrt : Sqrt
  Trigonometric Function : Trigonometry  Operator=asin
  Fs#_W : Outport
  Ms#_B : Outport  Port=2
  wires:
  Gain/1 -> Mux/1
  Product5/1 -> Product4/1
  Product4/1 -> Ms#_B/1
  Constant8/1 -> Product5/2
  Divide6/1 -> Product5/1  "M_s#"
  Add3/1 -> Fs#_W/1
  c_s#/1 -> Divide6/1
  Constant7/1 -> Divide6/2
  Add6/1 -> Divide6/3
  S_s#/1 -> Divide2/5, Divide5/5, Divide6/6
  rho/1 -> Divide2/3, Divide5/3, Divide6/4
  Dot Product1/1 -> Sqrt/1, Divide2/4, Divide5/4, Divide6/5
  Divide5/1 -> Gain/1  "D_s#"
  Constant6/1 -> Divide5/1
  Product3/1 -> Add6/2
  CM0_s#/1 -> Add6/1
  CMa_s#/1 -> Product3/1
  Constant5/1 -> Mux/3, Mux/2
  Add5/1 -> Divide5/2
  CD0_s#/1 -> Add5/1
  Product1/1 -> Add5/2
  Divide4/1 -> Add5/3
  e_s#/1 -> Divide4/3
  Constant4/1 -> Divide4/2
  Product2/1 -> Divide4/1
  CDa_s#/1 -> Product1/1
  Product/1 -> Product1/2
  Add4/1 -> Product/2, Product/1
  a0_s#/1 -> Add4/1
  Mux/1 -> Add3/1
  Divide3/1 -> Add3/2  "F_s#_Lonly"
  Divide2/1 -> Divide3/2  "L_s#"
  Constant3/1 -> Divide2/1
  Add2/1 -> Divide2/2
  CL0_s#/1 -> Add2/2
  Divide1/1 -> Add2/1, Product2/2, Product2/1  "CL_s#"
  Fcn/1 -> Divide1/2  "CLa_s#"
  AR_s#/1 -> Fcn/1, Divide4/4
  Add1/1 -> Divide1/1, Display1/1, Add4/2, Product3/2  "alpha_s#"
  i_s#/1 -> Add1/2
  Divide/1 -> Trigonometric Function/1
  Sqrt/1 -> MinMax/1
  MinMax/1 -> Divide/2
  Constant1/1 -> MinMax/2
  Dot Product/1 -> Divide/1
  n_s#/1 -> Dot Product/2, Divide3/1, Display/1, Product4/2
  v_B_BA/1 -> Dot Product/1, Dot Product1/2, Dot Product1/1
  Gain1/1 -> Add1/1
  Trigonometric Function/1 -> Gain1/1
  u_s#/1 -> Product6/1
  Su_S_ratio_s#/1 -> Product6/2
  dCL_du_s#/1 -> Product6/3
  Product6/1 -> Add2/3

== system Aircraft6dof_forTrimAndLin_ATT_wInputs/Equations Of Motion State Equations/QUAT2DCM/Subsystem ==
  normal(q) : Inport
  Demux : Demux
  Product{,1..3} (4 alike) : Product  RndMeth=Zero
  Sum : Sum  Inputs=++--
  A11 : Outport
  wires:
  Product3/1 -> Sum/1
  Demux/2 -> Product2/2, Product2/1
  Product1/1 -> Sum/3
  Demux/3 -> Product1/2, Product1/1
  Product2/1 -> Sum/2
  Sum/1 -> A11/1
  Product/1 -> Sum/4
  Demux/1 -> Product3/2, Product3/1
  normal(q)/1 -> Demux/1
  Demux/4 -> Product/2, Product/1

== system Aircraft6dof_forTrimAndLin_ATT_wInputs/Equations Of Motion State Equations/QUAT2DCM/Subsystem1 ==
  normal(q) : Inport
  Demux : Demux
  Gain : Gain  Gain=2
  Product2 : Product  RndMeth=Zero
  Product3 : Product  RndMeth=Zero
  Sum : Sum  Inputs=|++
  A12 : Outport
  wires:
  Product2/1 -> Sum/2
  Product3/1 -> Sum/1
  Sum/1 -> Gain/1
  Demux/1 -> Product3/2
  Demux/2 -> Product2/1
  Demux/4 -> Product3/1
  Demux/3 -> Product2/2
  normal(q)/1 -> Demux/1
  Gain/1 -> A12/1

== system Aircraft6dof_forTrimAndLin_ATT_wInputs/Equations Of Motion State Equations/QUAT2DCM/Subsystem2 ==
  normal(q) : Inport
  Demux : Demux
  Gain : Gain  Gain=2
  Product1 : Product  RndMeth=Zero
  Product2 : Product  RndMeth=Zero
  Sum : Sum  Inputs=|-+
  A13 : Outport
  wires:
  Demux/1 -> Product1/1
  Product1/1 -> Sum/1
  Product2/1 -> Sum/2
  Demux/4 -> Product2/2
  Demux/2 -> Product2/1
  Demux/3 -> Product1/2
  normal(q)/1 -> Demux/1
  Gain/1 -> A13/1
  Sum/1 -> Gain/1

== system Aircraft6dof_forTrimAndLin_ATT_wInputs/Equations Of Motion State Equations/QUAT2DCM/Subsystem3 ==
  normal(q) : Inport
  Demux : Demux
  Gain : Gain  Gain=2
  Product2 : Product  RndMeth=Zero
  Product3 : Product  RndMeth=Zero
  Sum : Sum  Inputs=|-+
  A21 : Outport
  wires:
  Gain/1 -> A21/1
  normal(q)/1 -> Demux/1
  Demux/3 -> Product2/2
  Demux/4 -> Product3/1
  Demux/2 -> Product2/1
  Demux/1 -> Product3/2
  Sum/1 -> Gain/1
  Product3/1 -> Sum/1
  Product2/1 -> Sum/2

== system Aircraft6dof_forTrimAndLin_ATT_wInputs/Equations Of Motion State Equations/QUAT2DCM/Subsystem4 ==
  normal(q) : Inport
  Demux : Demux
  Gain : Gain  Gain=2
  Product1 : Product  RndMeth=Zero
  Product2 : Product  RndMeth=Zero
  Sum : Sum  Inputs=|++
  A23 : Outport
  wires:
  Demux/4 -> Product2/2
  Product2/1 -> Sum/2
  Product1/1 -> Sum/1
  Sum/1 -> Gain/1
  Demux/1 -> Product1/1
  Demux/2 -> Product1/2
  Demux/3 -> Product2/1
  Gain/1 -> A23/1
  normal(q)/1 -> Demux/1
